simulink model "p2ctrl"  (Simulink 6.3)
settings: Solver=ode45  StartTime=0.0  StopTime=10.0  MaxStep=0.2  RelTol=1e-3
undefined symbols (not defined in the file or in its folder): FDab, planar2
libraries: simulink x4
settings Model: Creator=roy  LastModifiedBy=roy  ExtModeAutoUpdateStatusClock=off

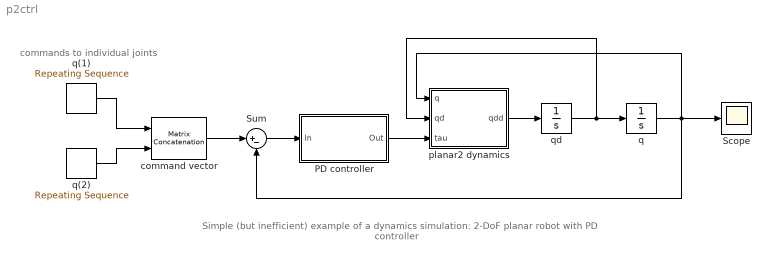
== system p2ctrl ==
  note: commands to
      | individual joints
  note: Simple (but inefficient) example of a dynamics simulation: 2-DoF planar robot with PD controller
  PD controller : Subsystem
  Scope : Scope
      settings: YMin=-0.5  YMax=2
  Sum : Sum  Inputs=|+-
  command vector : simulink/Math Operations/Matrix Concatenation  numInports=2  catMethod=Vertical
  planar2 dynamics : Subsystem
  q : Integrator  InitialCondition=[0;0]
  q(1) : simulink/Sources/Repeating Sequence  rep_seq_t=[0 1 2 3 4]  rep_seq_y=[0 1 1 0 0]
  q(2) : simulink/Sources/Repeating Sequence  rep_seq_t=[0 1 2 3 4]  rep_seq_y=[0 1.5 1.5 0 0]
  qd : Integrator  InitialCondition=[0;0]
  wires:
  planar2 dynamics/1(qdd) -> qd/1
  qd/1 -> q/1, planar2 dynamics/2(qd)
  q/1 -> Scope/1, planar2 dynamics/1(q), Sum/2
  PD controller/1(Out) -> planar2 dynamics/3(tau)
  Sum/1 -> PD controller/1(In)
  command vector/1 -> Sum/1
  q(2)/1 -> command vector/2
  q(1)/1 -> command vector/1

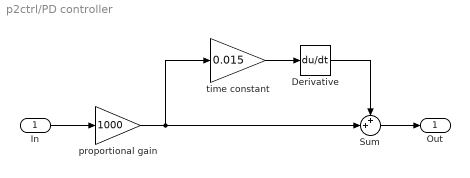
== system p2ctrl/PD controller ==
  In : Inport
  Derivative : Derivative
  Sum : Sum  Inputs=++|
  proportional gain : Gain  Gain=1000
  time constant : Gain  Gain=0.015
  Out : Outport
  wires:
  Sum/1 -> Out/1
  proportional gain/1 -> Sum/2, time constant/1
  In/1 -> proportional gain/1
  Derivative/1 -> Sum/1
  time constant/1 -> Derivative/1

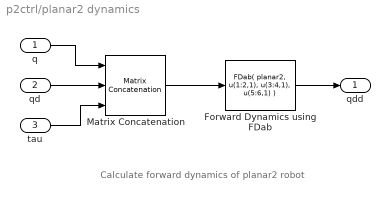
== system p2ctrl/planar2 dynamics ==
  note: Calculate forward dynamics of planar2 robot
  q : Inport
  qd : Inport  Port=2
  tau : Inport  Port=3
  Forward Dynamics using FDab : MATLABFcn  MATLABFcn=FDab( planar2, u(1:2,1), u(3:4,1), u(5:6,1) )  OutputDimensions=[2,1]  OutputSignalType=real  Output1D=off
  Matrix Concatenation : simulink/Math Operations/Matrix Concatenation  numInports=3  catMethod=Vertical
  qdd : Outport
  wires:
  qd/1 -> Matrix Concatenation/2
  tau/1 -> Matrix Concatenation/3
  q/1 -> Matrix Concatenation/1
  Matrix Concatenation/1 -> Forward Dynamics using FDab/1
  Forward Dynamics using FDab/1 -> qdd/1
